simulink model "shema"  (R2024b)
settings: Solver=VariableStepAuto  StartTime=0.0  StopTime=10  RelTol=1e-3
values from neighbouring files (symbols this model uses):
  f = 400    [dn_7.m]
  g = 9.82    [dn_7.m]
  l = 30    [dn_7.m]
  m_1 = 80    [dn_7.m]
  m_2 = 20    [dn_7.m]
settings Model: Creator=gaspers  LastModifiedBy=gaspers

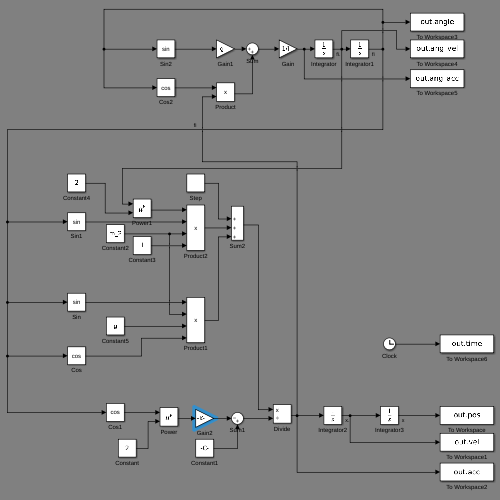
[thumbnail: Simulink's stored preview of the top-level diagram]
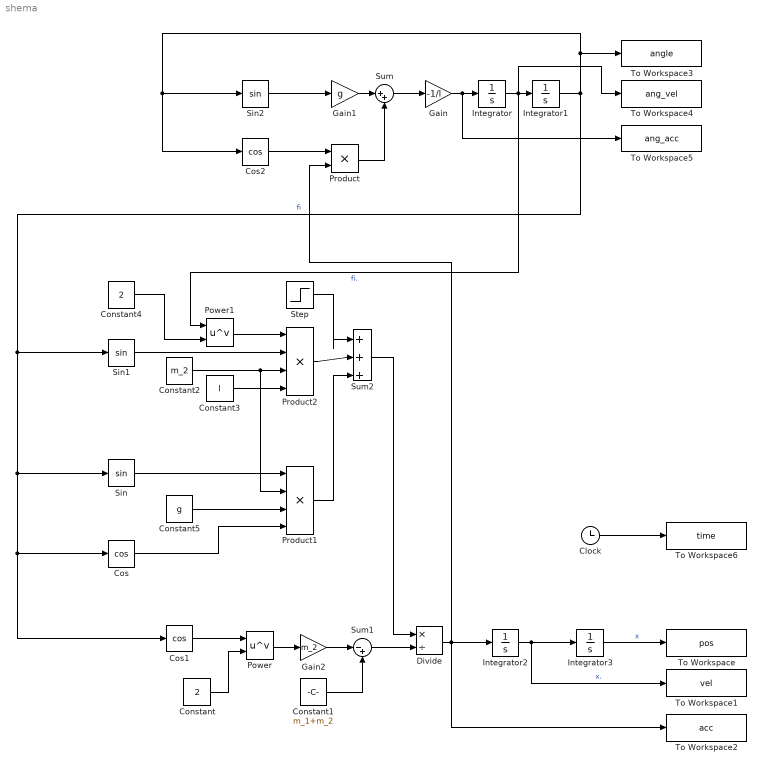
== system shema ==
  Clock : Clock
  Constant : Constant  Value=2
  Constant1 : Constant  Value=m_1+m_2
  Constant2 : Constant  Value=m_2
  Constant3 : Constant  Value=l
  Constant4 : Constant  Value=2
  Constant5 : Constant  Value=g
  Cos : Trigonometry  Operator=cos
  Cos1 : Trigonometry  Operator=cos
  Cos2 : Trigonometry  Operator=cos
  Divide : Product  Inputs=*/
  Gain : Gain  Gain=-1/l
  Gain1 : Gain  Gain=g
  Gain2 : Gain  Gain=m_2
  Integrator{,1..3} (4 alike) : Integrator
  Power : Math  Operator=pow
  Power1 : Math  Operator=pow
  Product : Product
  Product1 : Product  Inputs=4
  Product2 : Product  Inputs=4
  Sin : Trigonometry
  Sin1 : Trigonometry
  Sin2 : Trigonometry
  Step : Step  After=f  SampleTime=0
  Sum : Sum  Inputs=|++
  Sum1 : Sum  Inputs=|-+
  Sum2 : Sum  Inputs=|+++
  To Workspace : ToWorkspace  VariableName=pos  SampleTime=-1
  To Workspace1 : ToWorkspace  VariableName=vel  SampleTime=-1
  To Workspace2 : ToWorkspace  VariableName=acc  SampleTime=-1
  To Workspace3 : ToWorkspace  VariableName=angle  SampleTime=-1
  To Workspace4 : ToWorkspace  VariableName=ang_vel  SampleTime=-1
  To Workspace5 : ToWorkspace  VariableName=ang_acc  SampleTime=-1
  To Workspace6 : ToWorkspace  VariableName=time  SampleTime=-1
  wires:
  Integrator/1 -> Power1/1, To Workspace4/1, Integrator1/1  "fi."
  Integrator1/1 -> To Workspace3/1, Cos2/1, Sin2/1, Sin1/1, Sin/1, Cos1/1, Cos/1  "fi"
  Gain/1 -> To Workspace5/1, Integrator/1
  Sum/1 -> Gain/1
  Sin2/1 -> Gain1/1
  Gain1/1 -> Sum/1
  Cos2/1 -> Product/1
  Product/1 -> Sum/2
  Integrator2/1 -> To Workspace1/1, Integrator3/1  "x."
  Sum1/1 -> Divide/2
  Cos1/1 -> Power/1
  Power/1 -> Gain2/1
  Constant/1 -> Power/2
  Gain2/1 -> Sum1/1
  Constant1/1 -> Sum1/2
  Divide/1 -> To Workspace2/1, Product/2, Integrator2/1
  Step/1 -> Sum2/1
  Sum2/1 -> Divide/1
  Product2/1 -> Sum2/2
  Constant3/1 -> Product2/4
  Constant2/1 -> Product1/2, Product2/3
  Sin1/1 -> Product2/2
  Power1/1 -> Product2/1
  Constant4/1 -> Power1/2
  Cos/1 -> Product1/4
  Sin/1 -> Product1/1
  Constant5/1 -> Product1/3
  Product1/1 -> Sum2/3
  Integrator3/1 -> To Workspace/1  "x"
  Clock/1 -> To Workspace6/1
